simulink model "quantizer_ex"  (Simulink 7.2)
settings: Solver=ode45  StartTime=0.0  StopTime=.02  RelTol=1e-3
libraries: simulink x2, dspquant2 x1
settings Model: Creator=ahmed-salah  LastModifiedBy=ahmed-salah

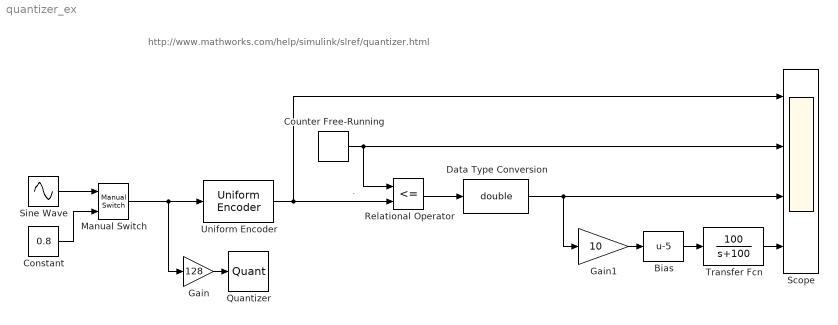
== system quantizer_ex ==
  note: http://www.mathworks.com/help/simulink/slref/quantizer.html
  note: .
  Bias : Bias  Bias=-5
  Constant : Constant  Value=0.8  OutDataType=sfix(16)  OutScaling=2^0
  Counter Free-Running : simulink/Sources/Counter Free-Running  SystemSampleTime=-1  NumBits=8  tsamp=1/1e6
  Data Type Conversion : DataTypeConversion  OutDataTypeMode=double  OutDataType=sfix(16)  OutScaling=2^0  OutDataTypeStr=double
  Gain : Gain  Gain=128  ParameterDataType=sfix(16)  ParameterScaling=2^0  OutDataType=sfix(16)  OutScaling=2^0
  Gain1 : Gain  Gain=10  ParameterDataType=sfix(16)  ParameterScaling=2^0  OutDataType=sfix(16)  OutScaling=2^0
  Manual Switch : simulink/Signal Routing/Manual Switch  SystemSampleTime=-1  sw=1  action=0  varsize=off
  Quantizer : Quantizer  QuantizationInterval=1  LinearizeAsGain=off  SampleTime=1/10e3
  Relational Operator : RelationalOperator  Operator=<=  LogicOutDataTypeMode=boolean  OutDataTypeStr=boolean  SampleTime=0
  Scope : Scope  NumInputPorts=4
      settings: YMin=0~0~-1~-5  YMax=275~275~1.5~5
  Sine Wave : Sin  Amplitude=1.2  Frequency=100*2*pi  SampleTime=0
  Transfer Fcn : TransferFcn  Numerator=[100]  Denominator="[1  100]"
  Uniform Encoder : dspquant2/Uniform Encoder  peak=1  bits=8  otype=Unsigned integer
  wires:
  Manual Switch/1 -> Uniform Encoder/1, Gain/1
  Uniform Encoder/1 -> Relational Operator/2, Scope/1
  Gain/1 -> Quantizer/1
  Relational Operator/1 -> Data Type Conversion/1
  Data Type Conversion/1 -> Gain1/1, Scope/3
  Counter Free-Running/1 -> Relational Operator/1, Scope/2
  Sine Wave/1 -> Manual Switch/1
  Constant/1 -> Manual Switch/2
  Gain1/1 -> Bias/1
  Bias/1 -> Transfer Fcn/1
  Transfer Fcn/1 -> Scope/4
